simulink model "problem9"  (R2020a)
settings: Solver=VariableStepAuto  StartTime=0.0  StopTime=10.0  RelTol=1e-3
model workspace (MAT data in the model file):
  Kd = Simulink.Parameter
  Kd.Value = 0.1
  Kd.DataType = 'auto'
  Kd.Dimensions = [1 1]
  Ki = Simulink.Parameter
  Ki.Value = 120
  Ki.DataType = 'auto'
  Ki.Dimensions = [1 1]
  Kp = Simulink.Parameter
  Kp.Value = 10
  Kp.DataType = 'auto'
  Kp.Dimensions = [1 1]
settings Model: Creator=Riyansh  LastModifiedBy=Riyansh

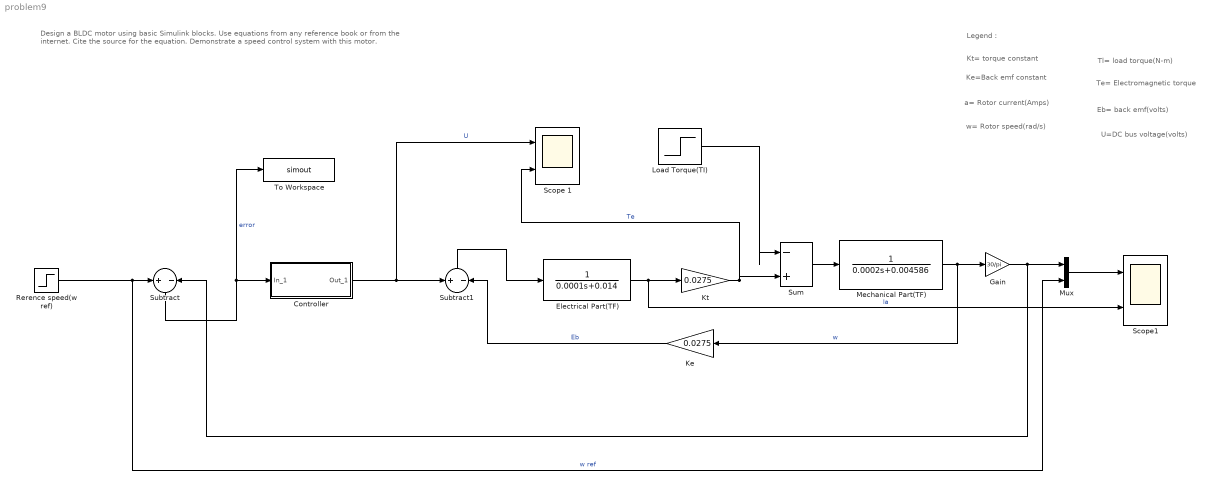
== system problem9 ==
  note: U=DC bus voltage(volts)
  note: Eb= back emf(volts)
  note: Te= Electromagnetic torque
  note: Tl= load torque(N-m)
  note: w= Rotor speed(rad/s)
  note: a= Rotor current(Amps)
  note: Ke=Back emf constant
  note: Kt= torque constant
  note: Legend :
  note: Design a BLDC motor using basic Simulink blocks. Use equations from any reference book or from the internet.
      | Cite the source for the equation. Demonstrate a speed control system with this motor.
  Controller : Subsystem
  Electrical Part(TF) : TransferFcn  Denominator=[0.0001 0.014]
  Gain : Gain  Gain=30/pi
  Ke : Gain  Gain=0.0275
  Kt : Gain  Gain=0.0275
  Load Torque(TI) : Step  Time=0.1  After=10  SampleTime=0
  Mechanical Part(TF) : TransferFcn  Denominator=[0.0002 0.004586]
  Mux : Mux  Inputs=2
  Rerence speed(w ref) : Step  Time=0  After=1500  SampleTime=0
  Scope 1 : Scope  NumInputPorts=2
  Scope1 : Scope  NumInputPorts=2
  Subtract : Sum  Inputs=+-
  Subtract1 : Sum  Inputs=+-
  Sum : Sum  Inputs=|-+
  To Workspace : ToWorkspace  VariableName=simout  SaveFormat=Timeseries  SampleTime=-1
  wires:
  Mechanical Part(TF)/1 -> Gain/1, Ke/1  "w"
  Rerence speed(w ref)/1 -> Mux/2, Subtract/1  "w ref"
  Gain/1 -> Subtract/2, Mux/1
  Electrical Part(TF)/1 -> Scope1/2, Kt/1  "la"
  Load Torque(TI)/1 -> Sum/1
  Ke/1 -> Subtract1/2  "Eb"
  Subtract1/1 -> Electrical Part(TF)/1
  Subtract/1 -> To Workspace/1, Controller/1(In_1)  "error"
  Sum/1 -> Mechanical Part(TF)/1
  Controller/1(Out_1) -> Scope 1/1, Subtract1/1  "U"
  Mux/1 -> Scope1/1
  Kt/1 -> Scope 1/2, Sum/2  "Te"

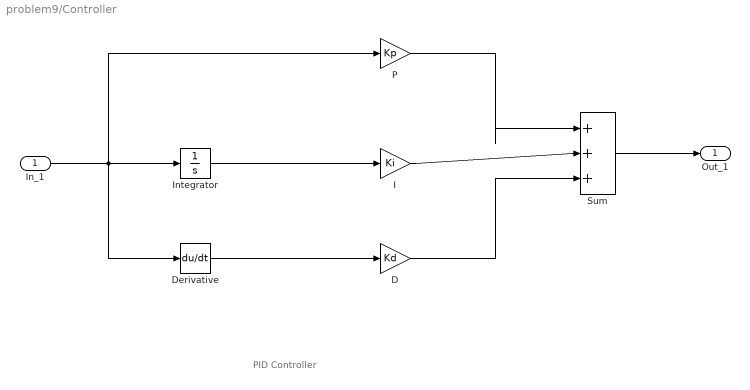
== system problem9/Controller ==
  note: PID Controller
  In_1 : Inport
  D : Gain  Gain=Kd
  Derivative : Derivative
  I : Gain  Gain=Ki
  Integrator : Integrator
  P : Gain  Gain=Kp
  Sum : Sum  Inputs=|+++
  Out_1 : Outport
  wires:
  In_1/1 -> Derivative/1, P/1, Integrator/1
  Derivative/1 -> D/1
  Integrator/1 -> I/1
  P/1 -> Sum/1
  I/1 -> Sum/2
  D/1 -> Sum/3
  Sum/1 -> Out_1/1
